simulink model "webcams"  (R2017a)
settings: Solver=VariableStepAuto  StartTime=0.0  StopTime=10.0  RelTol=1e-3
undefined symbols (not defined in the file or in its folder): Rec, SDTV
libraries: visionconversions x1, visionanalysis x1, dspvision x1
settings Model: Creator=ChiChaChai  LastModifiedBy=ChiChaChai

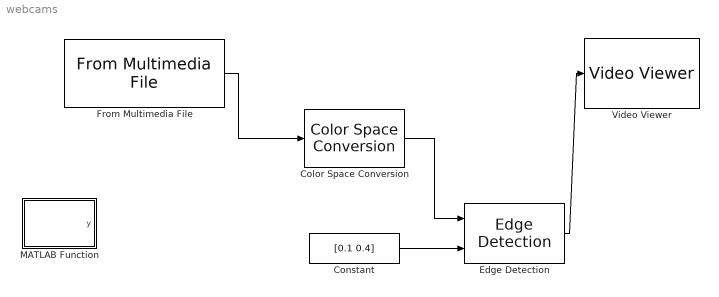
== system webcams ==
  Color Space Conversion : visionconversions/Color Space  Conversion  conversion=Obsolete  conversionActive=R'G'B' to intensity  wp_str=D65  rec=Rec. 601 (SDTV)  sys=1125/60/2:1  imagePorts=One multidimensional signal
      settings: SourceProductName=Computer Vision System Toolbox
  Constant : Constant  Value=[0.1 0.4]  OutDataTypeStr=single
  Edge Detection : visionanalysis/Edge Detection  method=Canny  outputType=Binary image  userDefinedThreshold=on  thresholdSource=Input port  threshold=20  thresholdTuning=4  edgeThinning=off  threshold_canny=[0.1 0.4]  autoPercent=70  sigma=1  prodOutputMode=Binary point scaling  prodOutputWordLength=32  prodOutputFracLength=8  roundingMode=Floor  overflowMode=off
      settings: SourceProductName=Computer Vision System Toolbox  SourceProductBaseCode=VP
  From Multimedia File : dspvision/From Multimedia File  inputFilename=C:\Users\ChiChaChai\Documents\AMAS 2017\SelfDrivingCar_with_MATLAB\challenge.mp4  loop=on  numPlays=inf  outputStreams=Video only  videoDataType=single  audioDataType=int16  inheritSampleTime=on  userDefinedSampleTime=1/30  noAudioOutput=off  isIntensityVideo=off  fourcc=RGB  colorVideoFormat=One multidimensional signal  outputEOF=off  dataOrg=Column-major  audioFrameSize=1024  computeAudioFrameSize=off  outSamplingMode=Sample based
      settings: SourceProductBaseCode=VP
  MATLAB Function : MATLAB Function  TreatAsAtomicUnit=on
  Video Viewer : VideoViewer  FigPos=[407.4 803.6 884 532.8]
  wires:
  From Multimedia File/1 -> Color Space Conversion/1
  Color Space Conversion/1 -> Edge Detection/1
  Edge Detection/1 -> Video Viewer/1
  Constant/1 -> Edge Detection/2

== matlab function webcams/MATLAB Function ==
  data: y output
function y = fcn()
y=0;
